simulink model "suspension"  (R2023a)
settings: Solver=VariableStepAuto  StartTime=0.0  StopTime=20  RelTol=1e-3
values from neighbouring files (symbols this model uses):
  c0 = 2050    [SYS_parameters.m]
  ks = 60000    [SYS_parameters.m]
  kt = 362000    [SYS_parameters.m]
  ms = 1173    [SYS_parameters.m]
  mu = 152.1    [SYS_parameters.m]
undefined symbols (not defined in the file or in its folder): K
libraries: dspsrcs4 x1
settings Model: Creator=huangdn  LastModifiedBy=Administrator
settings OptimizationCC: ReuseModelBlockBuffer=off

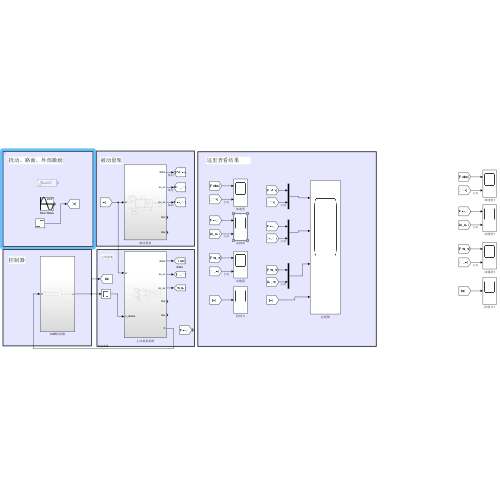
[thumbnail: Simulink's stored preview of the top-level diagram]
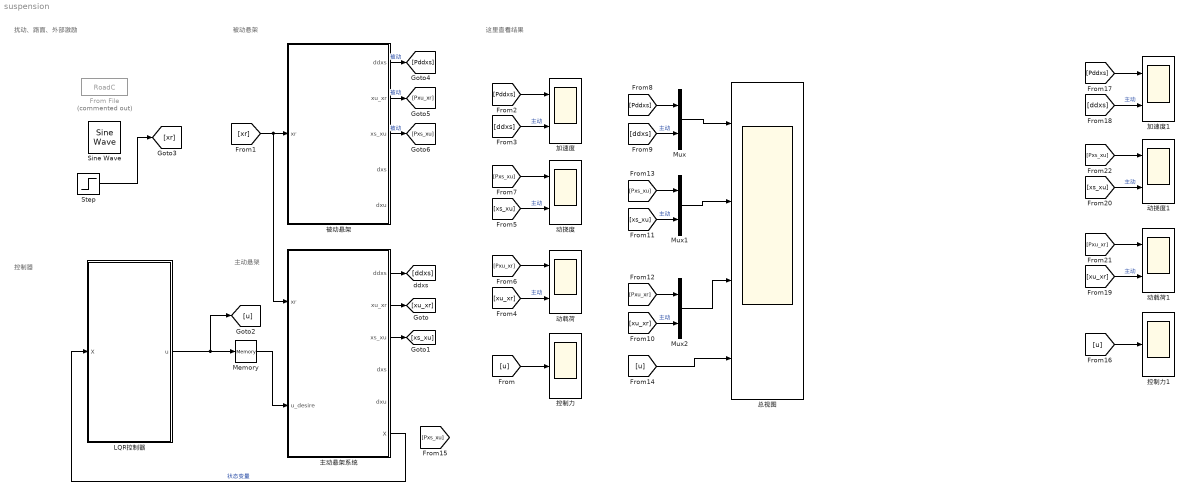
== system suspension ==
  note: 这里查看结果
  note: 主动悬架
  note: 被动悬架
  note: 控制器
  note: 扰动、路面、外部激励
  From File : FromFile  Commented=on  FileName=RoadC  SampleTime=0
  LQR控制器 : Subsystem
  Memory : Memory
  Mux : Mux  Inputs=2
  Mux1 : Mux  Inputs=2
  Mux2 : Mux  Inputs=2
  Sine Wave : dspsrcs4/Sine Wave  Amplitude=0.05  Frequency=1  Phase=0  SampleMode=Continuous  OutComplex=Real  CompMethod=Trigonometric fcn  TableSize=Speed  SampleTime=1/1000  SamplesPerFrame=1  ResetState=Restart at time zero  OutputFrames=off  dataType=double  wordLen=16  udDataType=sfix(16)  fracBitsMode=Best precision  numFracBits=15  OutDataTypeStr=double  LastOutDataTypeStr=double
  Step : Step  SampleTime=0
  主动悬架系统 : Subsystem
  加速度 : Scope  NumInputPorts=2
  加速度1 : Scope  NumInputPorts=2
  动挠度 : Scope  NumInputPorts=2
  动挠度1 : Scope  NumInputPorts=2
  动载荷 : Scope  NumInputPorts=2
  动载荷1 : Scope  NumInputPorts=2
  总视图 : Scope  NumInputPorts=4
  控制力 : Scope
  控制力1 : Scope
  被动悬架 : Subsystem
  wires:
  主动悬架系统/1(ddxs) -> [ddxs]
  主动悬架系统/2(xu_xr) -> [xu_xr]
  主动悬架系统/3(xs_xu) -> [xs_xu]
  [ddxs] -> 加速度/2  "主动"
  Memory/1 -> 主动悬架系统/2(u_desire)
  [xu_xr] -> 动载荷/2  "主动"
  [xs_xu] -> 动挠度/2  "主动"
  主动悬架系统/6(X) -> LQR控制器/1(X)  "状态变量"
  LQR控制器/1(u) -> [u], Memory/1
  [u] -> 控制力/1
  Mux1/1 -> 总视图/2
  Mux/1 -> 总视图/1
  Mux2/1 -> 总视图/3
  [xr] -> 主动悬架系统/1(xr), 被动悬架/1(xr)
  被动悬架/1(ddxs) -> [Pddxs]  "被动"
  被动悬架/2(xu_xr) -> [Pxu_xr]  "被动"
  被动悬架/3(xs_xu) -> [Pxs_xu]  "被动"
  [Pddxs] -> 加速度/1
  [Pxu_xr] -> 动载荷/1
  [Pxs_xu] -> 动挠度/1
  [Pddxs] -> Mux/1
  [ddxs] -> Mux/2  "主动"
  [Pxs_xu] -> Mux1/1
  [xs_xu] -> Mux1/2  "主动"
  [Pxu_xr] -> Mux2/1
  [xu_xr] -> Mux2/2  "主动"
  [u] -> 总视图/4
  Step/1 -> [xr]
  [xu_xr] -> 动载荷1/2  "主动"
  [Pxu_xr] -> 动载荷1/1
  [Pxs_xu] -> 动挠度1/1
  [xs_xu] -> 动挠度1/2  "主动"
  [u] -> 控制力1/1
  [Pddxs] -> 加速度1/1
  [ddxs] -> 加速度1/2  "主动"

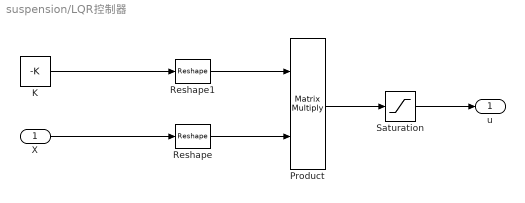
== system suspension/LQR控制器 ==
  X : Inport
  K : Constant  Value=-K
  Product : Product  Multiplication=Matrix(*)
  Reshape : Reshape  OutputDimensionality=Column vector (2-D)
  Reshape1 : Reshape  OutputDimensionality=Row vector (2-D)
  Saturation : Saturate  UpperLimit=2000  LowerLimit=-2000
  u : Outport
  wires:
  X/1 -> Reshape/1
  K/1 -> Reshape1/1
  Reshape/1 -> Product/2
  Product/1 -> Saturation/1
  Reshape1/1 -> Product/1
  Saturation/1 -> u/1

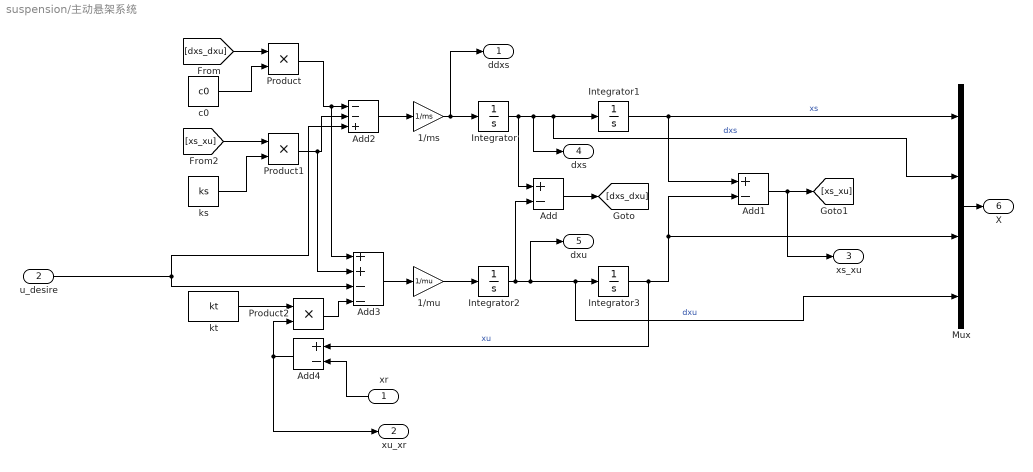
== system suspension/主动悬架系统 ==
  xr : Inport
  u_desire : Inport  Port=2
  1/ms : Gain  Gain=1/ms
  1/mu : Gain  Gain=1/mu
  Add : Sum  Inputs=+-
  Add1 : Sum  Inputs=+-
  Add2 : Sum  Inputs=--+
  Add3 : Sum  Inputs=++--
  Add4 : Sum  Inputs=+-
  Integrator{,1..3} (4 alike) : Integrator
  Mux : Mux
  Product : Product
  Product1 : Product
  Product2 : Product
  c0 : Constant  Value=c0
  ks : Constant  Value=ks
  kt : Constant  Value=kt
  ddxs : Outport
  xu_xr : Outport  Port=2
  xs_xu : Outport  Port=3
  dxs : Outport  Port=4
  dxu : Outport  Port=5
  X : Outport  Port=6
  wires:
  1/mu/1 -> Integrator2/1
  [xs_xu] -> Product1/1
  kt/1 -> Product2/1
  Add3/1 -> 1/mu/1
  Add2/1 -> 1/ms/1
  ks/1 -> Product1/2
  c0/1 -> Product/2
  Integrator3/1 -> Add4/1, Mux/3, Add1/2  "xu"
  Integrator1/1 -> Mux/1, Add1/1  "xs"
  xr/1 -> Add4/2
  Integrator2/1 -> Add/2, dxu/1, Mux/4, Integrator3/1  "dxu"
  Integrator/1 -> Mux/2, Integrator1/1, dxs/1, Add/1  "dxs"
  Product/1 -> Add3/1, Add2/1
  Add1/1 -> xs_xu/1, [xs_xu]
  [dxs_dxu] -> Product/1
  1/ms/1 -> ddxs/1, Integrator/1
  Add/1 -> [dxs_dxu]
  Add4/1 -> xu_xr/1, Product2/2
  Product1/1 -> Add3/2, Add2/2
  Product2/1 -> Add3/4
  Mux/1 -> X/1
  u_desire/1 -> Add3/3, Add2/3

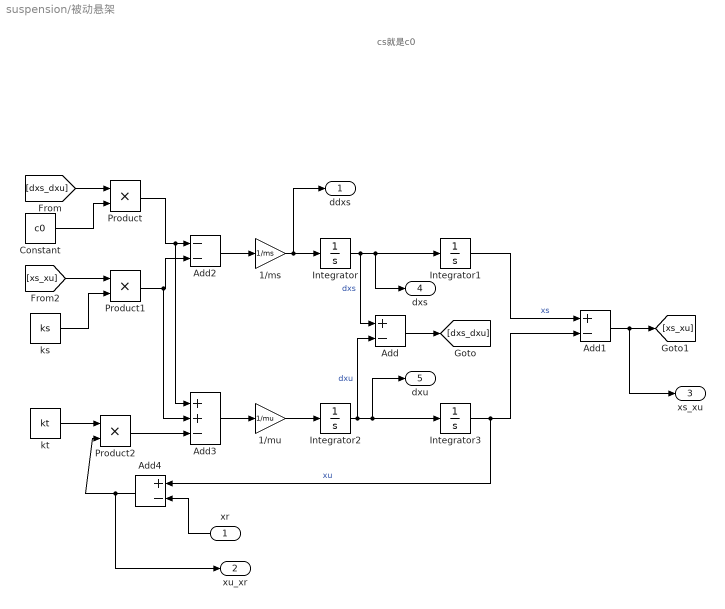
== system suspension/被动悬架 ==
  note: cs就是c0
  xr : Inport
  1/ms : Gain  Gain=1/ms
  1/mu : Gain  Gain=1/mu
  Add : Sum  Inputs=+-
  Add1 : Sum  Inputs=+-
  Add2 : Sum  Inputs=--
  Add3 : Sum  Inputs=++-
  Add4 : Sum  Inputs=+-
  Constant : Constant  Value=c0
  Integrator{,1..3} (4 alike) : Integrator
  Product : Product
  Product1 : Product
  Product2 : Product
  ks : Constant  Value=ks
  kt : Constant  Value=kt
  ddxs : Outport
  xu_xr : Outport  Port=2
  xs_xu : Outport  Port=3
  dxs : Outport  Port=4
  dxu : Outport  Port=5
  wires:
  Product1/1 -> Add2/2, Add3/2
  Add4/1 -> Product2/2, xu_xr/1
  Add/1 -> [dxs_dxu]
  1/ms/1 -> ddxs/1, Integrator/1
  [dxs_dxu] -> Product/1
  Add1/1 -> [xs_xu], xs_xu/1
  Product/1 -> Add2/1, Add3/1
  Integrator/1 -> Integrator1/1, dxs/1, Add/1  "dxs"
  Integrator2/1 -> Integrator3/1, dxu/1, Add/2  "dxu"
  xr/1 -> Add4/2
  Integrator1/1 -> Add1/1  "xs"
  Integrator3/1 -> Add1/2, Add4/1  "xu"
  Constant/1 -> Product/2
  ks/1 -> Product1/2
  Add2/1 -> 1/ms/1
  Add3/1 -> 1/mu/1
  kt/1 -> Product2/1
  [xs_xu] -> Product1/1
  Product2/1 -> Add3/3
  1/mu/1 -> Integrator2/1
